simulink model "Lighting"  (R2019a)
settings: Solver=VariableStepAuto  StartTime=0.0  StopTime=20  FixedStep=0.0001  RelTol=1e-3
libraries: ee_lib x32, nesl_utility x28, fl_lib x7, powerlib x2, re_lib x1, simulink x1
settings Model: Creator=CXJ889  LastModifiedBy=callu

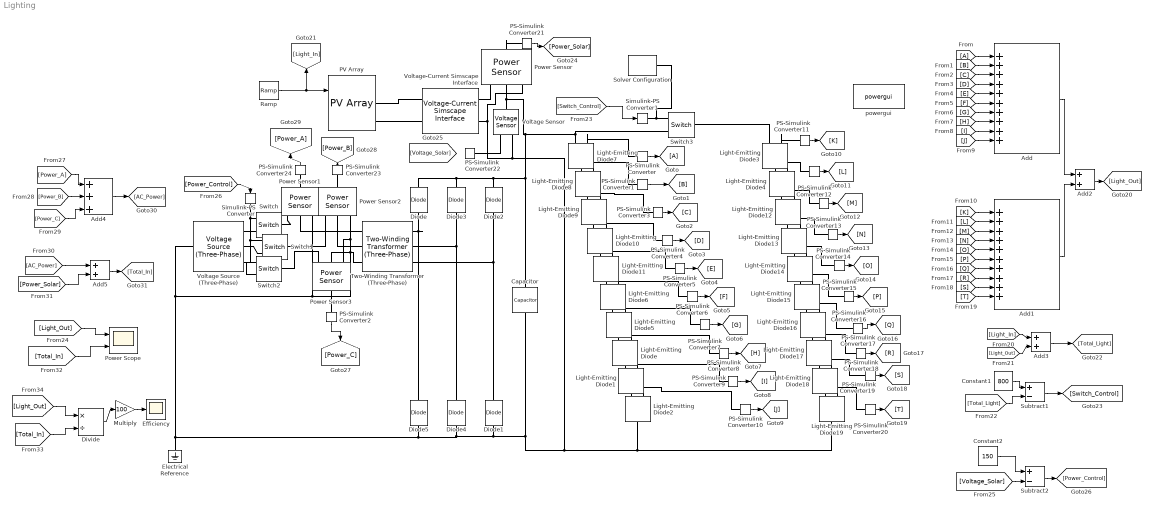
== system Lighting ==
  Add : Sum  Inputs=++++++++++
  Add1 : Sum  Inputs=++++++++++
  Add2 : Sum
  Add3 : Sum
  Add4 : Sum  Inputs=+++
  Add5 : Sum
  Capacitor : fl_lib/Electrical/Electrical Elements/Capacitor  c=0.5 F  r=1e-6 Ohm  g=0 1/Ohm  i_specify=off  i_priority=None  i=0 A  i_nominal_specify=off  i_nominal_unit=A  i_nominal_value=1  v_specify=off  v_priority=None  v=0 V  v_nominal_specify=off  v_nominal_unit=V  v_nominal_value=1  vc_specify=off  vc_priority=High  vc=0 V  vc_nominal_specify=off  vc_nominal_unit=V  vc_nominal_value=1
  Constant1 : Constant  Value=800
  Constant2 : Constant  Value=150
  Diode{,1..5} (6 alike) : ee_lib/Semiconductors & Converters/Diode  ModelType=ee.enum.diode.modelType.pwl  Vf=0.6 V  Ron=0.3 Ohm  Goff=1e-8 S  prmExp=ee.enum.diode.expParam.useTwo  I12=[.0137, .545] A  V12=[.6, .7] V  IS=1e-12 A  ec=1  I1=0.0137 A  V1=0.6 V  RS=0 Ohm  Tmeas=25 degC  N_series=1  N_parallel=1  Rz=0.3 Ohm  BV=inf V  C_param=ee.enum.diode.capParam.fixed  CJ=5 pF  CJ0=5 pF  VJ=1 V  Mgrad=0.5  Vvec=[.1, 10, 100] V  Cvec=[3.5, 1, .4] pF  FC=0.5  Q_param=ee.enum.diode.recoveryParam.off  iRM=-7.15 A  iF=4 A  didt=-750 A/us  trr_factor=3  trr=115 ns  Qrr=1500 s*uA  TT=50 ns  tau=100 ns  T_param=ee.enum.diode.temperatureParam.off  IS_T2=1.25e-7 A  I1_T2=0.245 A  V1_T2=0.5 V  Tmeas2=125 degC  EG_param=ee.enum.diode.egapParam.material_si  EG=1.11 eV  XTI_param=ee.enum.diode.xtiParam.pn  XTI=3  dBVdT=0 V/K  Tdevice=25 degC  i_specify=off  i_priority=None  i=0 A  i_nominal_specify=off  i_nominal_unit=A  i_nominal_value=1  v_specify=off  v_priority=None  v=0 V  v_nominal_specify=off  v_nominal_unit=V  v_nominal_value=1  i_capacitor_specify=off  i_capacitor_priority=None  i_capacitor=0 A  i_capacitor_nominal_specify=off  i_capacitor_nominal_unit=A  i_capacitor_nominal_value=1  v_capacitor_specify=off  v_capacitor_priority=None  v_capacitor=0 V  v_capacitor_nominal_specify=off  v_capacitor_nominal_unit=V  v_capacitor_nominal_value=1  power_dissipated_specify=off  power_dissipated_priority=None  power_dissipated=0 W  power_dissipated_nominal_specify=off  power_dissipated_nominal_unit=W  power_dissipated_nominal_value=1  Rth=[0, 10] K/W  thermal_mass_parameterization=ee.enum.thermalNetwork.timeconstant  thermal_mass=[0, 1] J/K  thermal_time_constant=[0, 10] s  thermal_mass_initial_temperatures=[25, 25] degC
      settings: SourceProductName=Simscape Electrical
  Divide : Product  Inputs=*/
  Efficiency : Scope
  Electrical Reference : fl_lib/Electrical/Electrical Elements/Electrical Reference
  Light-Emitting Diode{,1..19} (20 alike) : ee_lib/Sensors & Transducers/Light-Emitting Diode  Gain=0.005 W/A  prmExp=1  I12=[.0017, .003] A  V12=[.9, 1.05] V  IS=5e-5 A  ec=10  RS=0.1 Ohm  Tmeas=25 degC  C_param=1  CJ=20 pF  CJ0=20 pF  VJ=1 V  Mgrad=0.5  Vvec=[.1, 10, 100] V  Cvec=[15, 10, 2] pF  FC=0.5  T_param=1  IS_T2=1.8e-4 A  I1_T2=0.0034 A  V1_T2=1.05 V  Tmeas2=125 degC  EG_param=1  EG=1.11 eV  XTI_param=1  XTI=3  Tdevice=25 degC  i_capacitor_specify=off  i_capacitor_priority=High  i_capacitor=0 A  i_capacitor_nominal_specify=off  i_capacitor_nominal_unit=A  i_capacitor_nominal_value=1  v_capacitor_specify=off  v_capacitor_priority=None  v_capacitor=0 V  v_capacitor_nominal_specify=off  v_capacitor_nominal_unit=V  v_capacitor_nominal_value=1  Rth=[0, 10] K/W  thermal_mass_parameterization=1  thermal_mass=[0, 1] J/K  thermal_time_constant=[0, 10] s  thermal_mass_initial_temperatures=[25, 25] degC
      settings: SourceProductName=Simscape Electrical  SourceProductBaseCode=PS
  Multiply : Gain  Gain=100
  PS-Simulink Converter{,1..24} (25 alike) : nesl_utility/PS-Simulink Converter  PhysicalDomain=network_engine_domain  SubClassName=ps_output  LeftPortType=input  RightPortType=output  PseudoPeriodic=off  Frequencies=[]  Unit=1  AffineConversion=off
  PV Array : re_lib/Solar/PV Array  Npar=40  Nser=10  PlotType=array @ 1000 W/m2 & specified temperatures  S_vec="[ 1000  500  100 ]"  Temp_C_vec="[ 45 25  ]"  ModuleName=1Soltech 1STH-215-P  PlotWhenSelected=off  Pm=213.15  Ncell=60  Voc=36.3  Isc=7.84  Vm=29  Im=7.35  beta_Voc_pc=-0.36099  alpha_Isc_pc=0.102  beta_Voc=-0.13104  alpha_Isc=0.007997  IL=7.8649  I0=2.9259e-10  nI=0.98117  Rsh=313.3991  Rs=0.39383  BAL=off  Tc=1e-6  Tfilter=5e-5
      settings: SourceProductName=Simscape Electrical
  Power Scope : Scope  NumInputPorts=2
  Power Sensor{,1..3} (4 alike) : ee_lib/Sensors & Transducers/Power Sensor  measurement_type=1  averaging_period=1e-4 s
      settings: SourceProductName=Simscape Electrical  SourceProductBaseCode=PS
  Ramp : simulink/Sources/Ramp  slope=-10  start=0  InitialOutput=1000
  Simulink-PS Converter : nesl_utility/Simulink-PS Converter  PhysicalDomain=network_engine_domain  SubClassName=ps_input  LeftPortType=input  RightPortType=output  PseudoPeriodic=off  Frequencies=[]  NoiseDistribution=none  NoiseParameters=[]  Unit=1  AffineConversion=off  FilteringAndDerivatives=provide  SimscapeFilterOrder=1  InputFilterTimeConstant=0.001  UdotUserProvided=0
  Simulink-PS Converter1 : nesl_utility/Simulink-PS Converter  PhysicalDomain=network_engine_domain  SubClassName=ps_input  LeftPortType=input  RightPortType=output  PseudoPeriodic=off  Frequencies=[]  NoiseDistribution=none  NoiseParameters=[]  Unit=1  AffineConversion=off  FilteringAndDerivatives=provide  SimscapeFilterOrder=1  InputFilterTimeConstant=0.001  UdotUserProvided=0
  Solver Configuration : nesl_utility/Solver Configuration  PhysicalDomain=network_engine_domain  SubClassName=solver  LeftPortType=input  RightPortType=generic  Tones=[]  Harmonics=[]  SimulateNoise=off  Profile=off  UseLocalSampling=off  EnableSwitchedLinearOptims=on  FrequencyDomain=off  UseCCode=off  RelTol=0.001  AbsTol=1e-06  MinStep=1e-09  ToWorkspace=off  RevertToSquareIcSolve=off  NumHomotopyIterations=100  PhasorMode=off  PhasorModeNumHarmonics=1  DoDC=off  ResidualTolerance=1e-09  UseLocalSolver=off  LocalSolverChoice=NE_BACKWARD_EULER_ADVANCER  LocalSolverSampleTime=0.001  DoFixedCost=off  MaxNonlinIter=3  MaxModeIter=2  LinearAlgebra=auto  EquationFormulation=NE_TIME_EF  DelaysMemoryBudget=1024  AutomaticFiltering=on  FilteringTimeConstant=0.001  PartitionStorageMethod=AS_NEEDED  PartitionMemoryBudget=1024  PartitionMethod=ROBUST
  Subtract1 : Sum  Inputs=+-
  Subtract2 : Sum  Inputs=+-
  Switch{,1..3} (4 alike) : fl_lib/Electrical/Electrical Elements/Switch  R_closed=0.01 Ohm  G_open=1e-8 1/Ohm  Threshold=0  i_specify=off  i_priority=None  i=0 A  i_nominal_specify=off  i_nominal_unit=A  i_nominal_value=1  v_specify=off  v_priority=None  v=0 V  v_nominal_specify=off  v_nominal_unit=V  v_nominal_value=1
      settings: SourceProductName=Simscape
  Two-Winding Transformer (Three-Phase) : ee_lib/Passive/Transformers/Two-Winding Transformer (Three-Phase)  SRated=100e6 V*A  FRated=50 Hz  Winding1Connection=ee.enum.windingconnection.Y  VRated1=415 V  Winding2Connection=ee.enum.windingconnection.Y  VRated2=100 V  CoreType=ee.enum.coretype.threelimb  pu_Rw1=0.01  pu_Xl1=0.001  pu_Rw2=0.01  pu_Xl2=0.001  pu_Rm=500  pu_Xm=500  pu_X0=0.5  i1_specify=off  i1_priority=None  i1=[ 0 0 0 ] A  i1_nominal_specify=off  i1_nominal_unit=A  i1_nominal_value=1  i2_specify=off  i2_priority=None  i2=[ 0 0 0 ] A  i2_nominal_specify=off  i2_nominal_unit=A  i2_nominal_value=1  phi1_specify=off  phi1_priority=None  phi1=[ 0 0 0 ] Wb  phi1_nominal_specify=off  phi1_nominal_unit=Wb  phi1_nominal_value=1
      settings: SourceProductName=Simscape Electrical  SourceProductBaseCode=PS
  Voltage Source (Three-Phase) : ee_lib/Sources/Voltage Source (Three-Phase)  vline_rms=415 V  shift=0 deg  freq=50 Hz  impedance_option=1  SShortCircuit=1e6 V*A  XR=15  R=0.01 Ohm  L=3.97e-4 H  G_parasitic=0 1/Ohm  harmonic_option=0  harmonic_orders=[5, 7, 11, 13]  harmonic_ratios=[.1, .1, .1, .1]  I_specify=off  I_priority=None  I=[ 0 0 0 ] A  I_nominal_specify=off  I_nominal_unit=A  I_nominal_value=1
      settings: SourceProductName=Simscape Electrical  SourceProductBaseCode=PS  LogSimulationData=on
  Voltage Sensor : fl_lib/Electrical/Electrical Sensors/Voltage Sensor
  Voltage-Current Simscape Interface : powerlib/Interface Elements/Voltage-Current Simscape Interface  DFT=off  Fmode=Low pass filter (continuous)  T=1e-6  Ts=50e-6  i0=0  v0=0  Sd=Specialized Power Systems side  Measurements=off
      settings: SourceProductName=Simscape Electrical  SourceProductBaseCode=PS
  powergui : powerlib/powergui  Priority=1  SimulationMode=Continuous  SampleTime=50e-6  frequency=60  Iterations=50  frequencyindice=0  Pbase=100e6  ErrMax=1e-4  UnitsV=kV  UnitsW=MW  buscounter=0  FunctionMessages=off  echomessages=off  EnableUseOfTLC=off  CurrentSourceSwitches=off  DisableSnubberDevices=off  DisableRonSwitches=off  DisableVfSwitches=off  DisplayEquations=off  AutomaticDiscreteSolvers=off  SolverType=Tustin/Backward Euler (TBE)  Interpol=off  ExternalGateDelay=off  methode=off  Ts=100  x0status=blocks  SPID=on  SwTol=0  HookPort=off  NonlinearTolerance=0  nMaxIteration=15  ContinueOnMaxIteration=off  RestoreLinks=warning  ResistiveCurrentMeasurement=off  Frange=[0:2:500]  Ylog=off  Xlog=on  ShowGrid=off  save=off  variable=ZData  structure=0  ZoomFFT=off  StartTime=0.0  cycles=1  DisplayStyle=1  fundamental=60  FreqAxis=off  MaxFrequency=1000  frequencyindicesteady=1  RmsSteady=1  display=off
      settings: SourceProductName=Simscape Electrical
  wires:
  Ramp/1 -> PV Array/1, [Light_In]
  PS-Simulink Converter/1 -> [A]
  PS-Simulink Converter1/1 -> [B]
  PS-Simulink Converter3/1 -> [C]
  PS-Simulink Converter4/1 -> [D]
  PS-Simulink Converter5/1 -> [E]
  PS-Simulink Converter6/1 -> [F]
  PS-Simulink Converter7/1 -> [G]
  PS-Simulink Converter8/1 -> [H]
  PS-Simulink Converter9/1 -> [I]
  PS-Simulink Converter10/1 -> [J]
  [A] -> Add/1
  [C] -> Add/3
  [D] -> Add/4
  [B] -> Add/2
  [E] -> Add/5
  [F] -> Add/6
  [G] -> Add/7
  [H] -> Add/8
  [I] -> Add/9
  [J] -> Add/10
  PS-Simulink Converter11/1 -> [K]
  PS-Simulink Converter12/1 -> [L]
  PS-Simulink Converter13/1 -> [M]
  PS-Simulink Converter14/1 -> [N]
  PS-Simulink Converter15/1 -> [O]
  PS-Simulink Converter16/1 -> [P]
  PS-Simulink Converter17/1 -> [Q]
  PS-Simulink Converter18/1 -> [R]
  PS-Simulink Converter19/1 -> [S]
  PS-Simulink Converter20/1 -> [T]
  [K] -> Add1/1
  [L] -> Add1/2
  [M] -> Add1/3
  [N] -> Add1/4
  [O] -> Add1/5
  [P] -> Add1/6
  [Q] -> Add1/7
  [R] -> Add1/8
  [S] -> Add1/9
  [T] -> Add1/10
  Add/1 -> Add2/1
  Add1/1 -> Add2/2
  Add2/1 -> [Light_Out]
  [Light_In] -> Add3/1
  [Light_Out] -> Add3/2
  Add3/1 -> [Total_Light]
  Constant1/1 -> Subtract1/1
  [Total_Light] -> Subtract1/2
  Subtract1/1 -> [Switch_Control]
  [Switch_Control] -> Simulink-PS Converter1/1
  [Light_Out] -> Power Scope/1
  PS-Simulink Converter21/1 -> [Power_Solar]
  [Voltage_Solar] -> Subtract2/2
  Constant2/1 -> Subtract2/1
  Subtract2/1 -> [Power_Control]
  [Power_Control] -> Simulink-PS Converter/1
  PS-Simulink Converter2/1 -> [Power_C]
  PS-Simulink Converter23/1 -> [Power_B]
  PS-Simulink Converter24/1 -> [Power_A]
  [Power_A] -> Add4/1
  [Power_B] -> Add4/2
  [Power_C] -> Add4/3
  Add4/1 -> [AC_Power]
  [AC_Power] -> Add5/1
  [Power_Solar] -> Add5/2
  Add5/1 -> [Total_In]
  [Total_In] -> Power Scope/2
  [Total_In] -> Divide/2
  Multiply/1 -> Efficiency/1
  Divide/1 -> Multiply/1
  [Light_Out] -> Divide/1
  connections:
  Diode3/RConn1 -- Power Sensor/LConn2 -- Voltage Sensor/LConn1 -- Switch3/RConn2 -- Light-Emitting Diode7/LConn2 -- Capacitor/LConn1 -- Diode2/RConn1 -- Diode/RConn1
  Light-Emitting Diode2/LConn2 -- Light-Emitting Diode1/RConn1
  Light-Emitting Diode/RConn1 -- Light-Emitting Diode1/LConn2
  Voltage-Current Simscape Interface/LConn2 -- PV Array/RConn2
  PV Array/RConn1 -- Voltage-Current Simscape Interface/LConn1
  Light-Emitting Diode5/RConn1 -- Light-Emitting Diode/LConn2
  Light-Emitting Diode6/RConn1 -- Light-Emitting Diode5/LConn2
  Light-Emitting Diode11/RConn1 -- Light-Emitting Diode6/LConn2
  Light-Emitting Diode10/RConn1 -- Light-Emitting Diode11/LConn2
  Light-Emitting Diode9/RConn1 -- Light-Emitting Diode10/LConn2
  Light-Emitting Diode8/RConn1 -- Light-Emitting Diode9/LConn2
  Light-Emitting Diode7/RConn1 -- Light-Emitting Diode8/LConn2
  Power Sensor3/LConn2 -- Power Sensor3/LConn3 -- Power Sensor2/LConn3 -- Diode5/LConn1 -- Diode4/LConn1 -- Power Sensor/LConn3 -- Voltage-Current Simscape Interface/RConn2 -- Voltage Sensor/RConn2 -- Light-Emitting Diode19/RConn1 -- Light-Emitting Diode2/RConn1 -- Capacitor/RConn1 -- Diode1/LConn1 -- Electrical Reference/LConn1 -- Voltage Source (Three-Phase)/LConn1 -- Power Sensor1/LConn3 -- Two-Winding Transformer (Three-Phase)/LConn3
  Light-Emitting Diode4/LConn2 -- Light-Emitting Diode3/RConn1
  Light-Emitting Diode12/LConn2 -- Light-Emitting Diode4/RConn1
  Light-Emitting Diode13/LConn2 -- Light-Emitting Diode12/RConn1
  Light-Emitting Diode14/LConn2 -- Light-Emitting Diode13/RConn1
  Light-Emitting Diode15/LConn2 -- Light-Emitting Diode14/RConn1
  Light-Emitting Diode16/LConn2 -- Light-Emitting Diode15/RConn1
  Light-Emitting Diode17/LConn2 -- Light-Emitting Diode16/RConn1
  Light-Emitting Diode18/LConn2 -- Light-Emitting Diode17/RConn1
  Light-Emitting Diode19/LConn2 -- Light-Emitting Diode18/RConn1
  Diode5/RConn1 -- Two-Winding Transformer (Three-Phase)/RConn1 -- Diode/LConn1
  Diode4/RConn1 -- Two-Winding Transformer (Three-Phase)/RConn2 -- Diode3/LConn1
  Diode1/RConn1 -- Two-Winding Transformer (Three-Phase)/RConn3 -- Diode2/LConn1
  Light-Emitting Diode7/LConn1 -- PS-Simulink Converter/LConn1
  PS-Simulink Converter1/LConn1 -- Light-Emitting Diode8/LConn1
  PS-Simulink Converter3/LConn1 -- Light-Emitting Diode9/LConn1
  PS-Simulink Converter4/LConn1 -- Light-Emitting Diode10/LConn1
  PS-Simulink Converter5/LConn1 -- Light-Emitting Diode11/LConn1
  PS-Simulink Converter6/LConn1 -- Light-Emitting Diode6/LConn1
  PS-Simulink Converter7/LConn1 -- Light-Emitting Diode5/LConn1
  PS-Simulink Converter8/LConn1 -- Light-Emitting Diode/LConn1
  PS-Simulink Converter9/LConn1 -- Light-Emitting Diode1/LConn1
  PS-Simulink Converter10/LConn1 -- Light-Emitting Diode2/LConn1
  Light-Emitting Diode3/LConn1 -- PS-Simulink Converter11/LConn1
  PS-Simulink Converter12/LConn1 -- Light-Emitting Diode4/LConn1
  PS-Simulink Converter13/LConn1 -- Light-Emitting Diode12/LConn1
  PS-Simulink Converter14/LConn1 -- Light-Emitting Diode13/LConn1
  PS-Simulink Converter15/LConn1 -- Light-Emitting Diode14/LConn1
  PS-Simulink Converter16/LConn1 -- Light-Emitting Diode15/LConn1
  PS-Simulink Converter17/LConn1 -- Light-Emitting Diode16/LConn1
  PS-Simulink Converter18/LConn1 -- Light-Emitting Diode17/LConn1
  PS-Simulink Converter19/LConn1 -- Light-Emitting Diode18/LConn1
  PS-Simulink Converter20/LConn1 -- Light-Emitting Diode19/LConn1
  Light-Emitting Diode3/LConn2 -- Switch3/LConn1
  Simulink-PS Converter1/RConn1 -- Solver Configuration/RConn1 -- Switch3/RConn1
  Voltage-Current Simscape Interface/RConn1 -- Power Sensor/LConn1
  Power Sensor/RConn1 -- PS-Simulink Converter21/LConn1
  Voltage Sensor/RConn1 -- PS-Simulink Converter22/LConn1
  Switch/RConn2 -- Voltage Source (Three-Phase)/RConn1
  Simulink-PS Converter/RConn1 -- Switch2/RConn1 -- Switch1/RConn1 -- Switch/RConn1
  Voltage Source (Three-Phase)/RConn2 -- Switch1/RConn2
  Switch2/RConn2 -- Voltage Source (Three-Phase)/RConn3
  Switch/LConn1 -- Power Sensor1/LConn1
  Power Sensor1/LConn2 -- Two-Winding Transformer (Three-Phase)/LConn1
  Switch1/LConn1 -- Power Sensor2/LConn1
  Power Sensor2/LConn2 -- Two-Winding Transformer (Three-Phase)/LConn2
  Switch2/LConn1 -- Power Sensor3/LConn1
  PS-Simulink Converter2/LConn1 -- Power Sensor3/RConn1
  PS-Simulink Converter23/LConn1 -- Power Sensor2/RConn1
  PS-Simulink Converter24/LConn1 -- Power Sensor1/RConn1
